simulink model "Wipers_Model"  (R2025b)
settings: Solver=VariableStepAuto  StartTime=0.0  StopTime=10.0  RelTol=1e-3
libraries: simulink x21
settings Model: Creator=Sai Krishna  LastModifiedBy=Sai Krishna

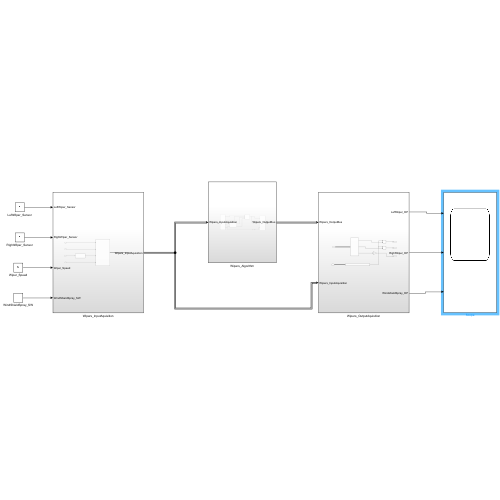
[thumbnail: Simulink's stored preview of the top-level diagram]
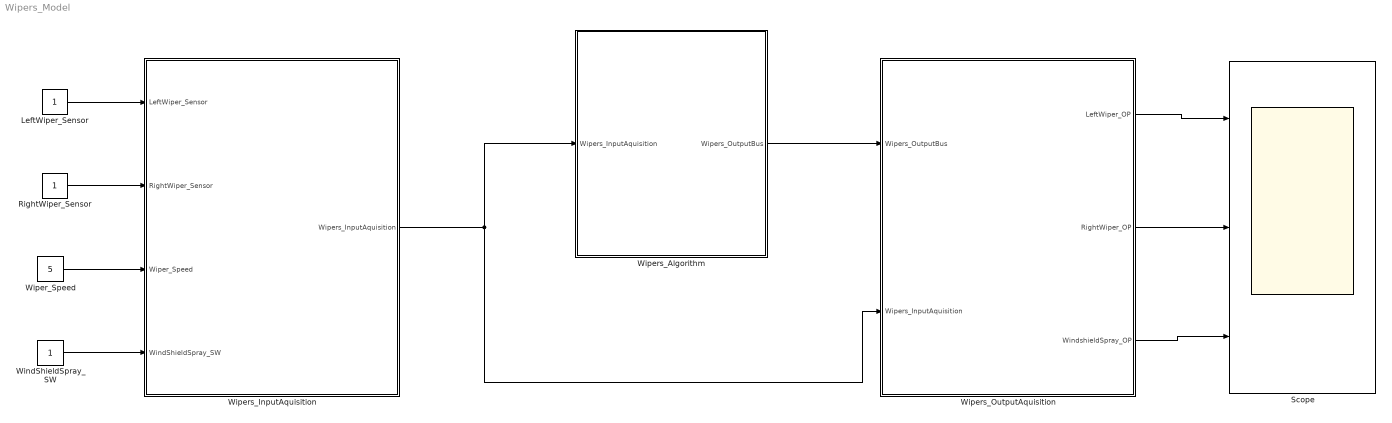
== system Wipers_Model ==
  LeftWiper_Sensor : Constant  OutDataTypeStr=boolean
  RightWiper_Sensor : Constant  OutDataTypeStr=boolean
  Scope : Scope  NumInputPorts=3
      settings: ActiveDisplayYMinimum=-10.606369631095394  ActiveDisplayYMaximum=38.196187845936258
  WindShieldSpray_SW : Constant  OutDataTypeStr=boolean
  Wiper_Speed : Constant  Value=5  OutDataTypeStr=double
  Wipers_Algorithm : Subsystem
  Wipers_InputAquisition : Subsystem
  Wipers_OutputAquisition : Subsystem
  wires:
  LeftWiper_Sensor/1 -> Wipers_InputAquisition/1(LeftWiper_Sensor)
  RightWiper_Sensor/1 -> Wipers_InputAquisition/2(RightWiper_Sensor)
  Wiper_Speed/1 -> Wipers_InputAquisition/3(Wiper_Speed)
  WindShieldSpray_SW/1 -> Wipers_InputAquisition/4(WindShieldSpray_SW)
  Wipers_InputAquisition/1(Wipers_InputAquisition) -> Wipers_OutputAquisition/2(Wipers_InputAquisition), Wipers_Algorithm/1(Wipers_InputAquisition)
  Wipers_Algorithm/1(Wipers_OutputBus) -> Wipers_OutputAquisition/1(Wipers_OutputBus)
  Wipers_OutputAquisition/2(RightWiper_OP) -> Scope/2
  Wipers_OutputAquisition/3(WindshieldSpray_OP) -> Scope/3
  Wipers_OutputAquisition/1(LeftWiper_OP) -> Scope/1

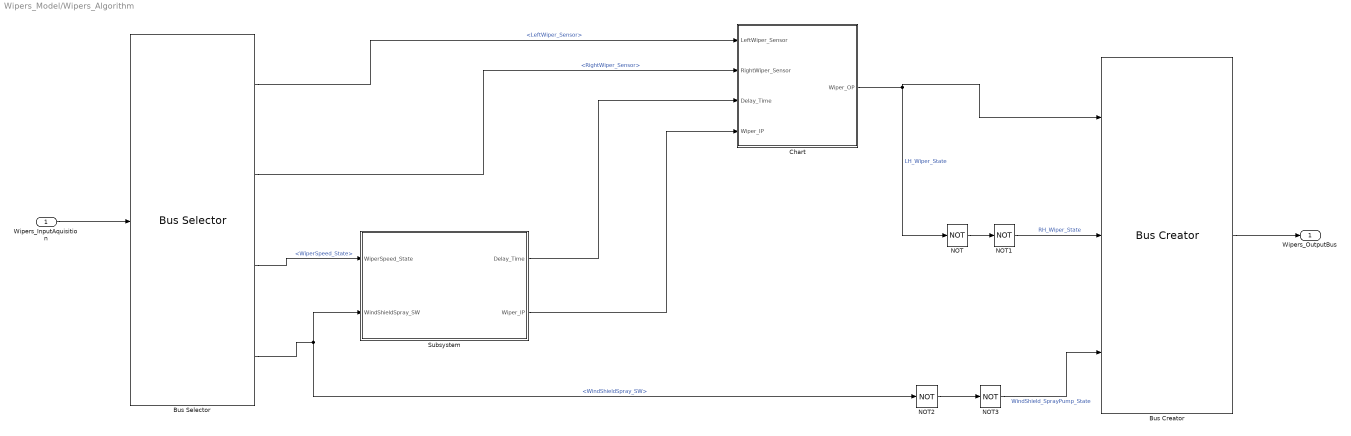
== system Wipers_Model/Wipers_Algorithm ==
  Wipers_InputAquisition : Inport  OutDataTypeStr=Bus: Wipers_InputBus
  Bus Creator : BusCreator  Inputs=3  OutDataTypeStr=Bus: Wipers_OutputBus
  Bus Selector : BusSelector  OutputSignals=LeftWiper_Sensor,RightWiper_Sensor,WiperSpeed_State,WindShieldSpray_SW
  Chart : Stateflow chart  TreatAsAtomicUnit=on
  NOT{,1..3} (4 alike) : Logic  Operator=NOT  IconShape=distinctive  AllPortsSameDT=off  OutDataTypeStr=boolean
  Subsystem : Subsystem
  Wipers_OutputBus : Outport  OutDataTypeStr=Bus: Wipers_OutputBus
  wires:
  Wipers_InputAquisition/1 -> Bus Selector/1
  Bus Creator/1 -> Wipers_OutputBus/1
  Bus Selector/1 -> Chart/1(LeftWiper_Sensor)  "<LeftWiper_Sensor>"
  Bus Selector/2 -> Chart/2(RightWiper_Sensor)  "<RightWiper_Sensor>"
  Bus Selector/3 -> Subsystem/1(WiperSpeed_State)  "<WiperSpeed_State>"
  Subsystem/1(Delay_Time) -> Chart/3(Delay_Time)
  Subsystem/2(Wiper_IP) -> Chart/4(Wiper_IP)
  Bus Selector/4 -> NOT2/1, Subsystem/2(WindShieldSpray_SW)  "<WindShieldSpray_SW>"
  Chart/1(Wiper_OP) -> Bus Creator/1, NOT/1  "LH_Wiper_State"
  NOT/1 -> NOT1/1
  NOT1/1 -> Bus Creator/2  "RH_Wiper_State"
  NOT2/1 -> NOT3/1
  NOT3/1 -> Bus Creator/3  "WindShield_SprayPump_State"

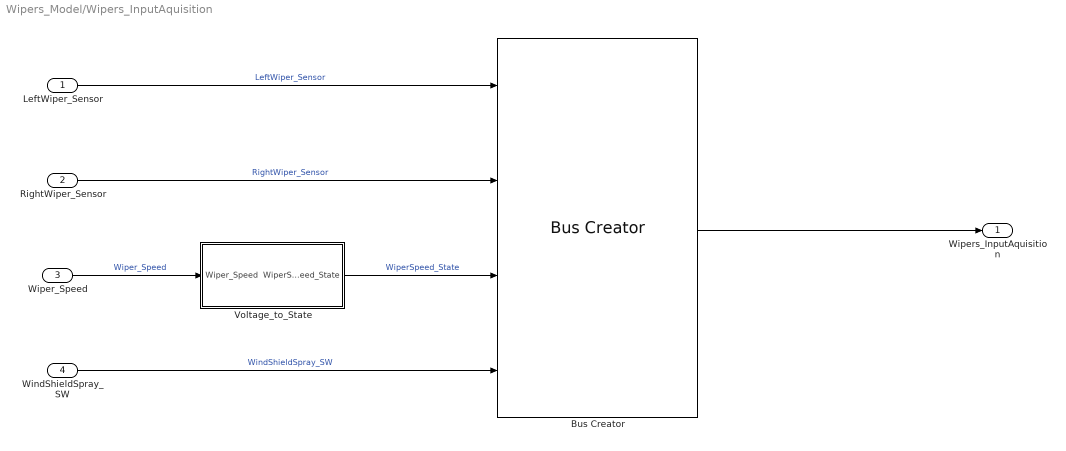
== system Wipers_Model/Wipers_InputAquisition ==
  LeftWiper_Sensor : Inport  OutDataTypeStr=boolean
  RightWiper_Sensor : Inport  Port=2  OutDataTypeStr=boolean
  Wiper_Speed : Inport  Port=3  OutDataTypeStr=double
  WindShieldSpray_SW : Inport  Port=4  OutDataTypeStr=boolean
  Bus Creator : BusCreator  Inputs=4  OutDataTypeStr=Bus: Wipers_InputBus
  Voltage_to_State : Subsystem
  Wipers_InputAquisition : Outport  OutDataTypeStr=Bus: Wipers_InputBus
  wires:
  LeftWiper_Sensor/1 -> Bus Creator/1  "LeftWiper_Sensor"
  RightWiper_Sensor/1 -> Bus Creator/2  "RightWiper_Sensor"
  WindShieldSpray_SW/1 -> Bus Creator/4  "WindShieldSpray_SW"
  Bus Creator/1 -> Wipers_InputAquisition/1
  Wiper_Speed/1 -> Voltage_to_State/1(Wiper_Speed)  "Wiper_Speed"
  Voltage_to_State/1(WiperSpeed_State) -> Bus Creator/3  "WiperSpeed_State"

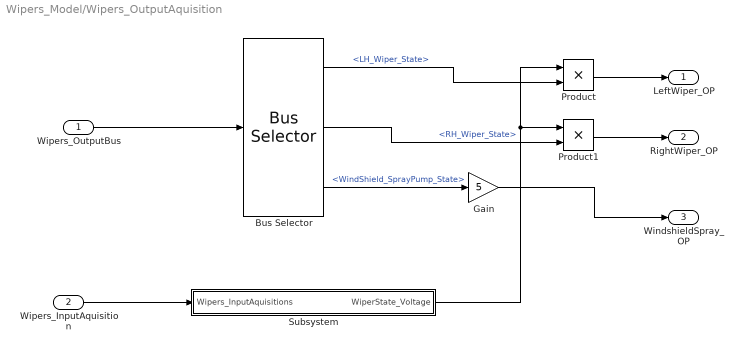
== system Wipers_Model/Wipers_OutputAquisition ==
  Wipers_OutputBus : Inport  OutDataTypeStr=Bus: Wipers_OutputBus
  Wipers_InputAquisition : Inport  Port=2  OutDataTypeStr=Bus: Wipers_InputBus
  Bus Selector : BusSelector  OutputSignals=LH_Wiper_State,RH_Wiper_State,WindShield_SprayPump_State
  Gain : Gain  Gain=5  OutDataTypeStr=double
  Product : Product  OutDataTypeStr=double
  Product1 : Product  OutDataTypeStr=double
  Subsystem : Subsystem
  LeftWiper_OP : Outport  OutDataTypeStr=double
  RightWiper_OP : Outport  Port=2  OutDataTypeStr=double
  WindshieldSpray_OP : Outport  Port=3  OutDataTypeStr=double
  wires:
  Wipers_OutputBus/1 -> Bus Selector/1
  Bus Selector/1 -> Product/2  "<LH_Wiper_State>"
  Bus Selector/2 -> Product1/2  "<RH_Wiper_State>"
  Bus Selector/3 -> Gain/1  "<WindShield_SprayPump_State>"
  Wipers_InputAquisition/1 -> Subsystem/1(Wipers_InputAquisitions)
  Subsystem/1(WiperState_Voltage) -> Product/1, Product1/1
  Product1/1 -> RightWiper_OP/1
  Product/1 -> LeftWiper_OP/1
  Gain/1 -> WindshieldSpray_OP/1

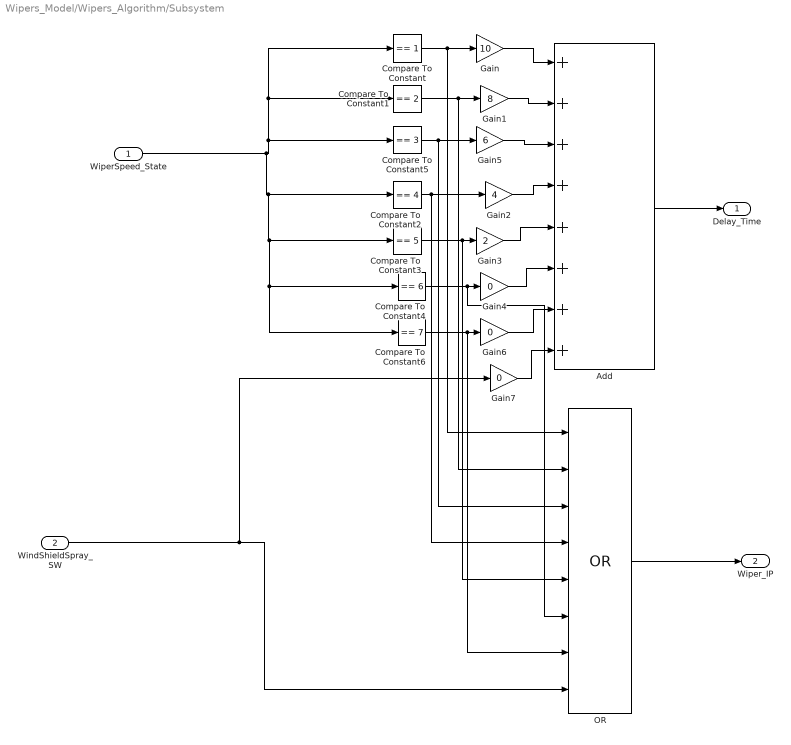
== system Wipers_Model/Wipers_Algorithm/Subsystem ==
  WiperSpeed_State : Inport
  WindShieldSpray_SW : Inport  Port=2
  Add : Sum  Inputs=++++++++
  Compare To Constant : simulink/Logic and Bit Operations/Compare To Constant  relop===  const=1  OutDataTypeStr=boolean
  Compare To Constant1 : simulink/Logic and Bit Operations/Compare To Constant  relop===  const=2  OutDataTypeStr=boolean
  Compare To Constant2 : simulink/Logic and Bit Operations/Compare To Constant  relop===  const=4  OutDataTypeStr=boolean
  Compare To Constant3 : simulink/Logic and Bit Operations/Compare To Constant  relop===  const=5  OutDataTypeStr=boolean
  Compare To Constant4 : simulink/Logic and Bit Operations/Compare To Constant  relop===  const=6  OutDataTypeStr=boolean
  Compare To Constant5 : simulink/Logic and Bit Operations/Compare To Constant  relop===  const=3  OutDataTypeStr=boolean
  Compare To Constant6 : simulink/Logic and Bit Operations/Compare To Constant  relop===  const=7  OutDataTypeStr=boolean
  Gain : Gain  Gain=10
  Gain1 : Gain  Gain=8
  Gain2 : Gain  Gain=4
  Gain3 : Gain  Gain=2
  Gain4 : Gain  Gain=0
  Gain5 : Gain  Gain=6
  Gain6 : Gain  Gain=0
  Gain7 : Gain  Gain=0
  OR : Logic  Operator=OR  Inputs=8  IconShape=distinctive  AllPortsSameDT=off  OutDataTypeStr=boolean
  Delay_Time : Outport
  Wiper_IP : Outport  Port=2
  wires:
  Compare To Constant/1 -> OR/1, Gain/1
  Compare To Constant1/1 -> OR/2, Gain1/1
  Compare To Constant2/1 -> OR/4, Gain2/1
  Compare To Constant3/1 -> OR/5, Gain3/1
  Compare To Constant4/1 -> OR/6, Gain4/1
  Compare To Constant5/1 -> OR/3, Gain5/1
  Compare To Constant6/1 -> OR/7, Gain6/1
  WiperSpeed_State/1 -> Compare To Constant6/1, Compare To Constant4/1, Compare To Constant3/1, Compare To Constant2/1, Compare To Constant/1, Compare To Constant1/1, Compare To Constant5/1
  Gain/1 -> Add/1
  Gain1/1 -> Add/2
  Gain5/1 -> Add/3
  Gain2/1 -> Add/4
  Gain3/1 -> Add/5
  Gain4/1 -> Add/6
  Gain6/1 -> Add/7
  Add/1 -> Delay_Time/1
  OR/1 -> Wiper_IP/1
  WindShieldSpray_SW/1 -> Gain7/1, OR/8
  Gain7/1 -> Add/8

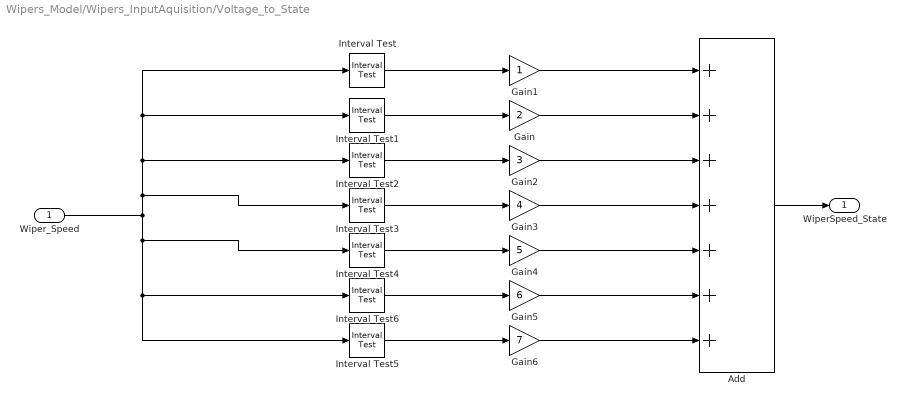
== system Wipers_Model/Wipers_InputAquisition/Voltage_to_State ==
  Wiper_Speed : Inport  OutDataTypeStr=double
  Add : Sum  Inputs=+++++++
  Gain : Gain  Gain=2  OutDataTypeStr=uint8
  Gain1 : Gain  OutDataTypeStr=uint8
  Gain2 : Gain  Gain=3  OutDataTypeStr=uint8
  Gain3 : Gain  Gain=4  OutDataTypeStr=uint8
  Gain4 : Gain  Gain=5  OutDataTypeStr=uint8
  Gain5 : Gain  Gain=6  OutDataTypeStr=uint8
  Gain6 : Gain  Gain=7  OutDataTypeStr=uint8
  Interval Test : simulink/Logic and Bit Operations/Interval Test  IntervalClosedRight=on  uplimit=1  IntervalClosedLeft=on  lowlimit=0.2  OutDataTypeStr=boolean
  Interval Test1 : simulink/Logic and Bit Operations/Interval Test  IntervalClosedRight=on  uplimit=2  IntervalClosedLeft=on  lowlimit=1.2  OutDataTypeStr=boolean
  Interval Test2 : simulink/Logic and Bit Operations/Interval Test  IntervalClosedRight=on  uplimit=3  IntervalClosedLeft=on  lowlimit=2.2  OutDataTypeStr=boolean
  Interval Test3 : simulink/Logic and Bit Operations/Interval Test  IntervalClosedRight=on  uplimit=4  IntervalClosedLeft=on  lowlimit=3.2  OutDataTypeStr=boolean
  Interval Test4 : simulink/Logic and Bit Operations/Interval Test  IntervalClosedRight=on  uplimit=5  IntervalClosedLeft=on  lowlimit=4.2  OutDataTypeStr=boolean
  Interval Test5 : simulink/Logic and Bit Operations/Interval Test  IntervalClosedRight=on  uplimit=7  IntervalClosedLeft=on  lowlimit=6.2  OutDataTypeStr=boolean
  Interval Test6 : simulink/Logic and Bit Operations/Interval Test  IntervalClosedRight=on  uplimit=6  IntervalClosedLeft=on  lowlimit=5.2  OutDataTypeStr=boolean
  WiperSpeed_State : Outport
  wires:
  Interval Test/1 -> Gain1/1
  Gain1/1 -> Add/1
  Gain/1 -> Add/2
  Gain2/1 -> Add/3
  Gain3/1 -> Add/4
  Gain4/1 -> Add/5
  Gain5/1 -> Add/6
  Gain6/1 -> Add/7
  Interval Test1/1 -> Gain/1
  Interval Test2/1 -> Gain2/1
  Interval Test3/1 -> Gain3/1
  Interval Test4/1 -> Gain4/1
  Interval Test6/1 -> Gain5/1
  Interval Test5/1 -> Gain6/1
  Wiper_Speed/1 -> Interval Test/1, Interval Test1/1, Interval Test2/1, Interval Test3/1, Interval Test5/1, Interval Test6/1, Interval Test4/1
  Add/1 -> WiperSpeed_State/1

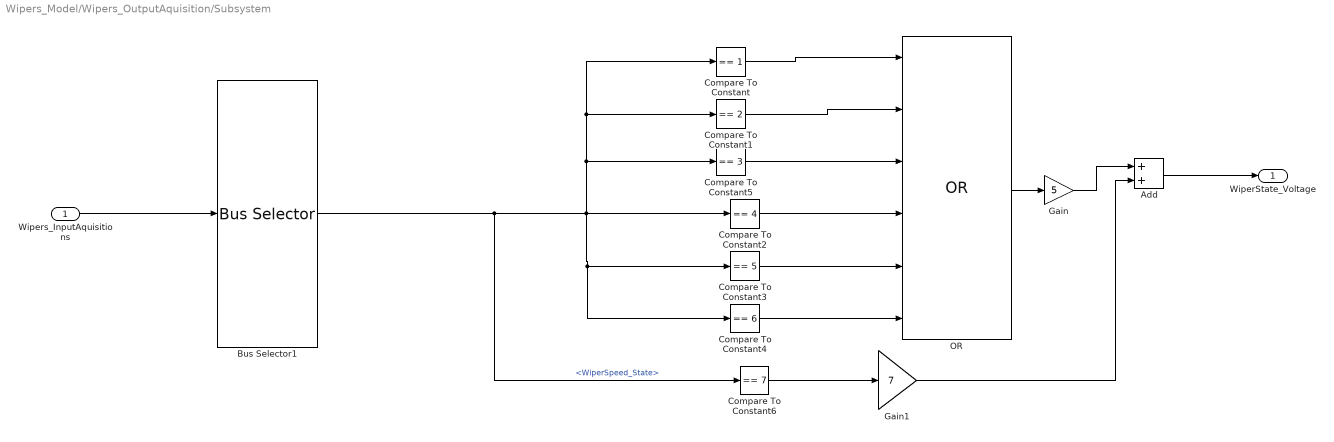
== system Wipers_Model/Wipers_OutputAquisition/Subsystem ==
  Wipers_InputAquisitions : Inport  OutDataTypeStr=Bus: Wipers_InputBus
  Add : Sum
  Bus Selector1 : BusSelector  OutputSignals=WiperSpeed_State
  Compare To Constant : simulink/Logic and Bit Operations/Compare To Constant  relop===  const=1  OutDataTypeStr=boolean
  Compare To Constant1 : simulink/Logic and Bit Operations/Compare To Constant  relop===  const=2  OutDataTypeStr=boolean
  Compare To Constant2 : simulink/Logic and Bit Operations/Compare To Constant  relop===  const=4  OutDataTypeStr=boolean
  Compare To Constant3 : simulink/Logic and Bit Operations/Compare To Constant  relop===  const=5  OutDataTypeStr=boolean
  Compare To Constant4 : simulink/Logic and Bit Operations/Compare To Constant  relop===  const=6  OutDataTypeStr=boolean
  Compare To Constant5 : simulink/Logic and Bit Operations/Compare To Constant  relop===  const=3  OutDataTypeStr=boolean
  Compare To Constant6 : simulink/Logic and Bit Operations/Compare To Constant  relop===  const=7  OutDataTypeStr=boolean
  Gain : Gain  Gain=5  OutDataTypeStr=double
  Gain1 : Gain  Gain=7  OutDataTypeStr=double
  OR : Logic  Operator=OR  Inputs=6  AllPortsSameDT=off  OutDataTypeStr=boolean
  WiperState_Voltage : Outport
  wires:
  Bus Selector1/1 -> Compare To Constant6/1, Compare To Constant/1, Compare To Constant1/1, Compare To Constant5/1, Compare To Constant4/1, Compare To Constant3/1, Compare To Constant2/1  "<WiperSpeed_State>"
  Compare To Constant3/1 -> OR/5
  Compare To Constant5/1 -> OR/3
  Gain/1 -> Add/1
  Compare To Constant1/1 -> OR/2
  Compare To Constant6/1 -> Gain1/1
  Wipers_InputAquisitions/1 -> Bus Selector1/1
  Compare To Constant/1 -> OR/1
  Compare To Constant2/1 -> OR/4
  Compare To Constant4/1 -> OR/6
  Gain1/1 -> Add/2
  OR/1 -> Gain/1
  Add/1 -> WiperState_Voltage/1

== stateflow chart Wipers_Model/Wipers_Algorithm/Chart ==
  state OFF_
    Wiper_OP=false;
  state ON_
    Wiper_OP=true;
  state WAIT_
    Wiper_OP=false;
  (default) -> OFF_
  OFF_ -> ON_ : [LeftWiper_Sensor==true && RightWiper_Sensor==true && Wiper_IP==true]
  WAIT_ -> ON_ [order 1] : [after(Delay_Time, sec) && Wiper_IP==true]
  ON_ -> WAIT_ : [LeftWiper_Sensor==true && RightWiper_Sensor==true]
  WAIT_ -> OFF_ [order 2] : [Wiper_IP==false]
  data: LeftWiper_Sensor input; RightWiper_Sensor input; Delay_Time input; Wiper_IP input; Wiper_OP output
